simulink model "TestSegmentCorde"  (R2019b)
settings: Solver=VariableStepAuto  StartTime=0.0  StopTime=10.0  RelTol=1e-3
settings Model: Creator=maxim  LastModifiedBy=maxim

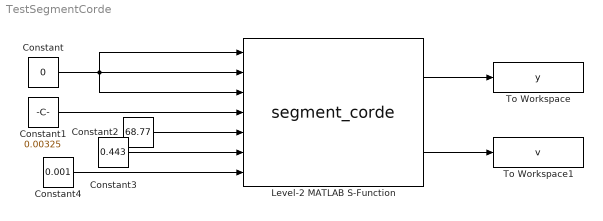
== system TestSegmentCorde ==
  Constant : Constant  Value=0
  Constant1 : Constant  Value=0.00325
  Constant2 : Constant  Value=68.77
  Constant3 : Constant  Value=0.443
  Constant4 : Constant  Value=0.001
  Level-2 MATLAB S-Function : M-S-Function  FunctionName=segment_corde
  To Workspace : ToWorkspace  VariableName=y  SaveFormat=Timeseries  SampleTime=-1
  To Workspace1 : ToWorkspace  VariableName=v  SaveFormat=Timeseries  SampleTime=-1
  wires:
  Constant/1 -> Level-2 MATLAB S-Function/1, Level-2 MATLAB S-Function/3, Level-2 MATLAB S-Function/2
  Constant1/1 -> Level-2 MATLAB S-Function/4
  Constant4/1 -> Level-2 MATLAB S-Function/7
  Constant3/1 -> Level-2 MATLAB S-Function/6
  Constant2/1 -> Level-2 MATLAB S-Function/5
  Level-2 MATLAB S-Function/2 -> To Workspace1/1
  Level-2 MATLAB S-Function/1 -> To Workspace/1
